simulink library "MotionPlanner_Library"  (R2025b)
settings: Solver=VariableStepAuto  StartTime=0.0  StopTime=10.0  RelTol=1e-3
values from neighbouring files (symbols this model uses):
  structMotionPlannerOut = struct()    [MotionPlanner_CreateExternalData.m]    (also in MotionPlanner_ExternalData.sldd = 0.0
                        0.0
                    
       )
undefined symbols (not defined in the file or in its folder): enable, finalPose, initialStateAndInput, originLLA, reset, samplingBoxCenterPose, samplingBoxDimension, sequentialPlanner, timestamp, verticesStaticObstacles
libraries: AVE_Library x7, MPSV x4, simulink x3, GenericTarget x1, simulink_extras x1
settings Model: Creator=damerius  LastModifiedBy=Scythe

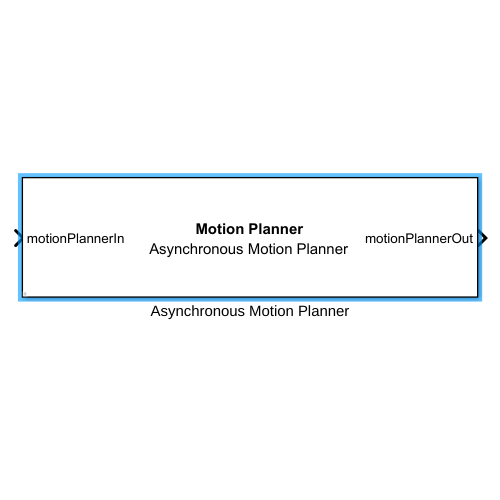
[thumbnail: Simulink's stored preview of the top-level diagram]
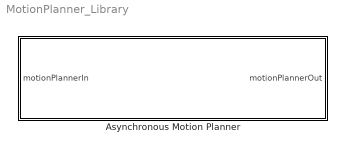
== system MotionPlanner_Library ==
  Asynchronous Motion Planner : Subsystem  mask{priorityWorkerThread=40, mpsvCPUCoresToUse=int32(0:7), sampletime=-1}
      mask prompts: priorityWorkerThread "Worker thread priority (1: low, 99: high):"; mpsvCPUCoresToUse "CPU cores on which the thread is eligible to run, e.g. [0,1,2,3] ([] to ignore):"; sampletime "Sample time (-1 for inherited):"
      mask help: Solves the motion planning problem in an asynchronous manner using parallel computing. The whole planner runs in a separate worker thread. Each time this block is executed, it passes data to the worker thread and fetches the latest results from it.
      mask DialogControl DescGroupVar Prompt: Asynchronous Motion Planner
      mask Display:
      | % Get dimension of block
      | pos = get_param(gcb, 'Position');
      | width = pos(3) - pos(1);
      | height = pos(4) - pos(2);
      | 
      | % Block title
      | text(0.5*width,0.5*height, '{\bfMotion Planner}','horizontalAlignment','center','verticalAlignment','bottom','texmode','on');
      | text(0.5*width,0.5*height, 'Asynchronous Motion Planner','horizontalAlignment','center','verticalAlignment','top','texmode','on');

== system MotionPlanner_Library/Asynchronous Motion Planner ==
  motionPlannerIn : Inport  OutDataTypeStr=Bus: busMotionPlannerIn  SampleTime=sampletime
  Asynchronous Motion Planner : Subsystem  TreatAsAtomicUnit=on
  Bus Selector : BusSelector  OutputSignals=parameter
  Planning Problem Generator : Subsystem
  Unit Delay : UnitDelay  SampleTime=sampletime  HasFrameUpgradeWarning=on
  check for automatic reset : Subsystem
  make output struct : Subsystem
  motionPlannerOut : Outport  OutDataTypeStr=Bus: busMotionPlannerOut  SampleTime=sampletime
  wires:
  make output struct/1(output) -> motionPlannerOut/1
  check for automatic reset/1(resetPlanner) -> Asynchronous Motion Planner/3(resetPlanner)
  Planning Problem Generator/1(planningProblem) -> Asynchronous Motion Planner/1(planningProblem)
  Asynchronous Motion Planner/1(motionPlanner) -> Unit Delay/1, make output struct/1(motionPlanner)
  Unit Delay/1 -> check for automatic reset/2(previousMotionPlanner)
  motionPlannerIn/1 -> check for automatic reset/1(input), Bus Selector/1, Planning Problem Generator/1(input)
  Bus Selector/1 -> Asynchronous Motion Planner/2(inputParameter)  "<parameter>"

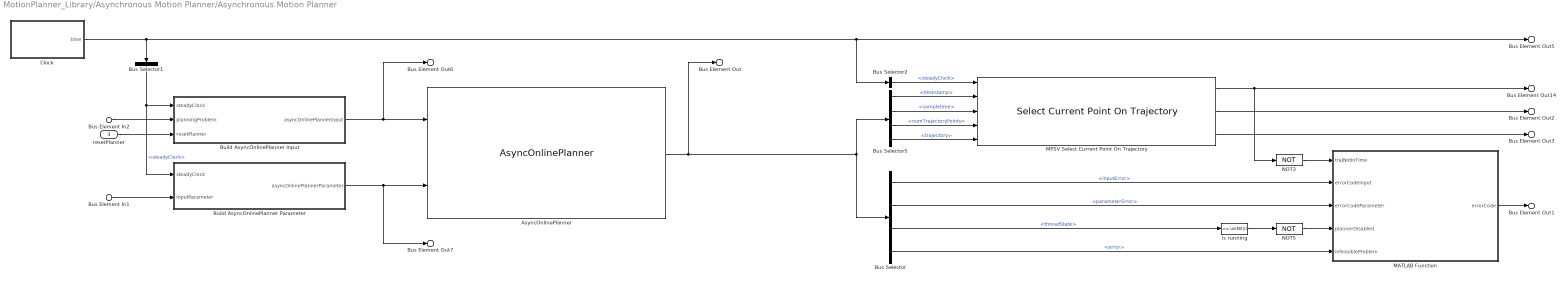
== system MotionPlanner_Library/Asynchronous Motion Planner/Asynchronous Motion Planner ==
  Bus Element In2 : Inport  PortName=planningProblem
  Bus Element In1 : Inport  Port=2  PortName=inputParameter
  resetPlanner : Inport  Port=3
  AsyncOnlinePlanner : MPSV/AsyncOnlinePlanner  pathMaxNumNodes=200  pathMaxNumSamples=1000000  motionMaxNumNodes=200  motionMaxNumSamples=1000000  threadPriority=priorityWorkerThread  cpuCoreIDs=mpsvCPUCoresToUse  ompNumThreads=numel(mpsvCPUCoresToUse) - 1  ompDynamic=0
      settings: SourceProductName=MPSV - Motion Planner for Surface Vehicles
  Build AsyncOnlinePlanner Input : Subsystem  Priority=2  TreatAsAtomicUnit=on
  Build AsyncOnlinePlanner Parameter : Subsystem  Priority=3  TreatAsAtomicUnit=on
  Bus Selector : BusSelector  OutputSignals=inputError,parameterError,threadState,error
  Bus Selector1 : BusSelector  OutputSignals=steadyClock
  Bus Selector2 : BusSelector  OutputSignals=steadyClock
  Bus Selector5 : BusSelector  OutputSignals=timestamp,sampletime,numTrajectoryPoints,trajectory
  Clock : Subsystem  Priority=1  TreatAsAtomicUnit=on  SystemSampleTime=sampletime
  MATLAB Function : MATLAB Function  TreatAsAtomicUnit=on
  MPSV Select Current Point On Trajectory : MPSV/Select Current Point On Trajectory
      settings: SourceProductName=MPSV - Motion Planner for Surface Vehicles
  NOT3 : Logic  Operator=NOT  AllPortsSameDT=off  OutDataTypeStr=boolean
  NOT5 : Logic  Operator=NOT  AllPortsSameDT=off  OutDataTypeStr=boolean
  is running : simulink/Logic and Bit Operations/Compare To Constant  relop===  const=uint8(2)  OutDataTypeStr=boolean
  Bus Element Out5 : Outport  PortName=motionPlanner  Element=time
  Bus Element Out : Outport  PortName=motionPlanner  Element=asyncOnlinePlannerOutput
  Bus Element Out14 : Outport  PortName=motionPlanner  Element=trajectoryPointSelector.success
  Bus Element Out2 : Outport  PortName=motionPlanner  Element=trajectoryPointSelector.currentPoint
  Bus Element Out3 : Outport  PortName=motionPlanner  Element=trajectoryPointSelector.remainingTrajectoryDuration
  Bus Element Out6 : Outport  PortName=motionPlanner  Element=asyncOnlinePlannerInput
  Bus Element Out7 : Outport  PortName=motionPlanner  Element=asyncOnlinePlannerParameter
  Bus Element Out1 : Outport  PortName=motionPlanner  Element=errorCode
  wires:
  MATLAB Function/1(errorCode) -> Bus Element Out1/1
  NOT3/1 -> MATLAB Function/1(trajNotInTime)
  Bus Selector/2 -> MATLAB Function/3(errorCodeParameter)  "<parameterError>"
  Bus Selector/1 -> MATLAB Function/2(errorCodeInput)  "<inputError>"
  resetPlanner/1 -> Build AsyncOnlinePlanner Input/3(resetPlanner)
  Bus Selector/4 -> MATLAB Function/5(infeasibleProblem)  "<error>"
  Bus Selector/3 -> is running/1  "<threadState>"
  Build AsyncOnlinePlanner Input/1(asyncOnlinePlannerInput) -> Bus Element Out6/1, AsyncOnlinePlanner/1
  AsyncOnlinePlanner/1 -> Bus Element Out/1, Bus Selector/1, Bus Selector5/1
  Bus Selector5/3 -> MPSV Select Current Point On Trajectory/4  "<numTrajectoryPoints>"
  Bus Selector5/1 -> MPSV Select Current Point On Trajectory/2  "<timestamp>"
  Bus Selector5/4 -> MPSV Select Current Point On Trajectory/5  "<trajectory>"
  Build AsyncOnlinePlanner Parameter/1(asyncOnlinePlannerParameter) -> Bus Element Out7/1, AsyncOnlinePlanner/2
  Bus Selector5/2 -> MPSV Select Current Point On Trajectory/3  "<sampletime>"
  MPSV Select Current Point On Trajectory/1 -> NOT3/1, Bus Element Out14/1
  MPSV Select Current Point On Trajectory/2 -> Bus Element Out2/1
  MPSV Select Current Point On Trajectory/3 -> Bus Element Out3/1
  Bus Element In2/1 -> Build AsyncOnlinePlanner Input/2(planningProblem)
  Bus Element In1/1 -> Build AsyncOnlinePlanner Parameter/2(inputParameter)
  is running/1 -> NOT5/1
  NOT5/1 -> MATLAB Function/4(plannerDisabled)
  Clock/1(time) -> Bus Selector2/1, Bus Element Out5/1, Bus Selector1/1
  Bus Selector1/1 -> Build AsyncOnlinePlanner Input/1(steadyClock), Build AsyncOnlinePlanner Parameter/1(steadyClock)  "<steadyClock>"
  Bus Selector2/1 -> MPSV Select Current Point On Trajectory/1  "<steadyClock>"

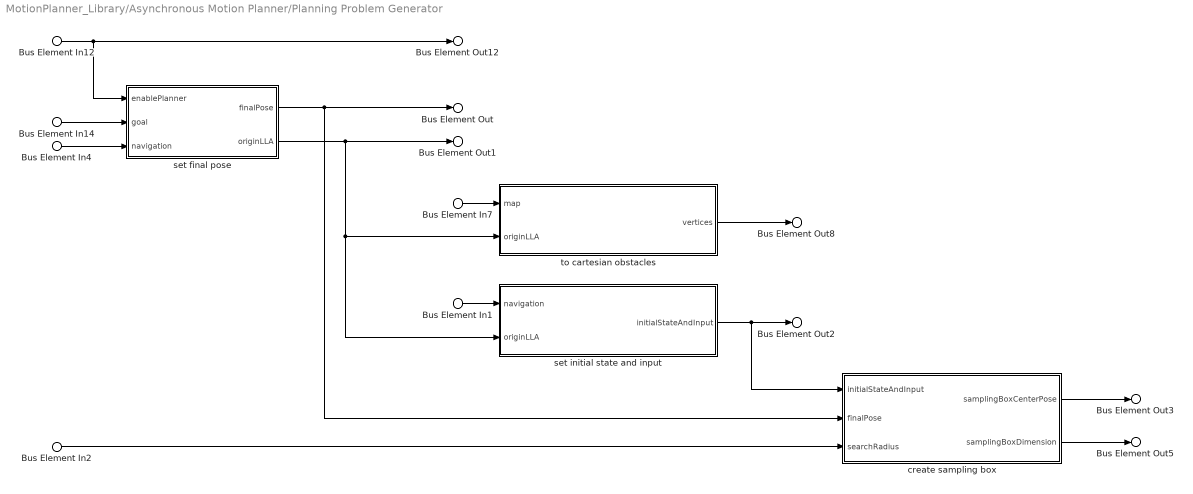
== system MotionPlanner_Library/Asynchronous Motion Planner/Planning Problem Generator ==
  Bus Element In14 : Inport  PortName=input  Element=goal
  Bus Element In7 : Inport  PortName=input  Element=map
  Bus Element In12 : Inport  PortName=input  Element=enablePlanner
  Bus Element In4 : Inport  PortName=input  Element=navigation
  Bus Element In1 : Inport  PortName=input  Element=navigation
  Bus Element In2 : Inport  PortName=input  Element=parameter.searchRadius
  create sampling box : Subsystem
  set final pose : Subsystem
  set initial state and input : Subsystem
  to cartesian obstacles : Subsystem
  Bus Element Out12 : Outport  PortName=planningProblem  Element=enablePlanner
  Bus Element Out1 : Outport  PortName=planningProblem  Element=originLLA
  Bus Element Out2 : Outport  PortName=planningProblem  Element=initialStateAndInput
  Bus Element Out : Outport  PortName=planningProblem  Element=finalPose
  Bus Element Out3 : Outport  PortName=planningProblem  Element=samplingBoxCenterPose
  Bus Element Out5 : Outport  PortName=planningProblem  Element=samplingBoxDimension
  Bus Element Out8 : Outport  PortName=planningProblem  Element=staticObstacles.vertices
  wires:
  Bus Element In12/1 -> Bus Element Out12/1, set final pose/1(enablePlanner)
  to cartesian obstacles/1(vertices) -> Bus Element Out8/1
  Bus Element In7/1 -> to cartesian obstacles/1(map)
  create sampling box/2(samplingBoxDimension) -> Bus Element Out5/1
  create sampling box/1(samplingBoxCenterPose) -> Bus Element Out3/1
  Bus Element In2/1 -> create sampling box/3(searchRadius)
  set initial state and input/1(initialStateAndInput) -> create sampling box/1(initialStateAndInput), Bus Element Out2/1
  set final pose/2(originLLA) -> Bus Element Out1/1, set initial state and input/2(originLLA), to cartesian obstacles/2(originLLA)
  set final pose/1(finalPose) -> Bus Element Out/1, create sampling box/2(finalPose)
  Bus Element In14/1 -> set final pose/2(goal)
  Bus Element In4/1 -> set final pose/3(navigation)
  Bus Element In1/1 -> set initial state and input/1(navigation)

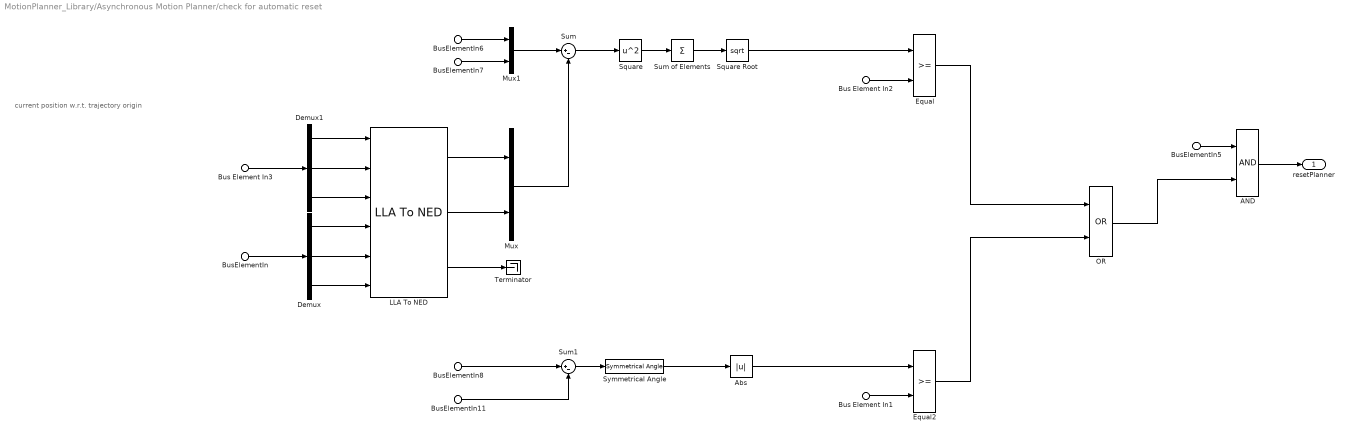
== system MotionPlanner_Library/Asynchronous Motion Planner/check for automatic reset ==
  note: current position w.r.t. trajectory origin
  Bus Element In3 : Inport  PortName=input  Element=navigation.positionLLA
  BusElementIn11 : Inport  PortName=input  Element=navigation.orientationYaw
  Bus Element In2 : Inport  PortName=input  Element=maxDeviationToReset.position
  Bus Element In1 : Inport  PortName=input  Element=maxDeviationToReset.heading
  BusElementIn : Inport  Port=2  PortName=previousMotionPlanner  Element=asyncOnlinePlannerOutput.originLLA
  BusElementIn5 : Inport  Port=2  PortName=previousMotionPlanner  Element=trajectoryPointSelector.success
  BusElementIn6 : Inport  Port=2  PortName=previousMotionPlanner  Element=trajectoryPointSelector.currentPoint.stateInterpolated.positionNorth
  BusElementIn7 : Inport  Port=2  PortName=previousMotionPlanner  Element=trajectoryPointSelector.currentPoint.stateInterpolated.positionEast
  BusElementIn8 : Inport  Port=2  PortName=previousMotionPlanner  Element=trajectoryPointSelector.currentPoint.stateInterpolated.orientationYaw
  AND : Logic  AllPortsSameDT=off  OutDataTypeStr=boolean
  Abs : Abs  SaturateOnIntegerOverflow=off
  Demux : Demux  Outputs=3
  Demux1 : Demux  Outputs=3
  Equal : RelationalOperator  OutDataTypeStr=boolean  RndMeth=Simplest  InputSameDT=off
  Equal2 : RelationalOperator  OutDataTypeStr=boolean  RndMeth=Simplest  InputSameDT=off
  LLA To NED : AVE_Library/Essential/Transformation/LLA To NED
      settings: SourceProductName=AVE - Autonomous Vehicle Control Toolbox
  Mux : Mux  Inputs=2
  Mux1 : Mux  Inputs=2
  OR : Logic  Operator=OR  AllPortsSameDT=off  OutDataTypeStr=boolean
  Square : Math  Operator=square
  Square Root : Sqrt
  Sum : Sum  Inputs=|+-
  Sum of Elements : Sum  Inputs=+
  Sum1 : Sum  Inputs=|+-
  Symmetrical Angle : AVE_Library/Essential/Symmetrical Angle
      settings: SourceProductName=AVE - Autonomous Vehicle Control Toolbox
  Terminator : Terminator
  resetPlanner : Outport
  wires:
  Demux1/3 -> LLA To NED/3
  Demux1/2 -> LLA To NED/2
  Demux1/1 -> LLA To NED/1
  Bus Element In3/1 -> Demux1/1
  BusElementIn/1 -> Demux/1
  Demux/1 -> LLA To NED/4
  Demux/2 -> LLA To NED/5
  Demux/3 -> LLA To NED/6
  LLA To NED/3 -> Terminator/1
  LLA To NED/2 -> Mux/2
  LLA To NED/1 -> Mux/1
  BusElementIn6/1 -> Mux1/1
  BusElementIn7/1 -> Mux1/2
  Mux1/1 -> Sum/1
  Mux/1 -> Sum/2
  Sum/1 -> Square/1
  Square/1 -> Sum of Elements/1
  Sum of Elements/1 -> Square Root/1
  BusElementIn8/1 -> Sum1/1
  BusElementIn11/1 -> Sum1/2
  Sum1/1 -> Symmetrical Angle/1
  Symmetrical Angle/1 -> Abs/1
  BusElementIn5/1 -> AND/1
  AND/1 -> resetPlanner/1
  OR/1 -> AND/2
  Square Root/1 -> Equal/1
  Bus Element In2/1 -> Equal/2
  Abs/1 -> Equal2/1
  Bus Element In1/1 -> Equal2/2
  Equal/1 -> OR/1
  Equal2/1 -> OR/2

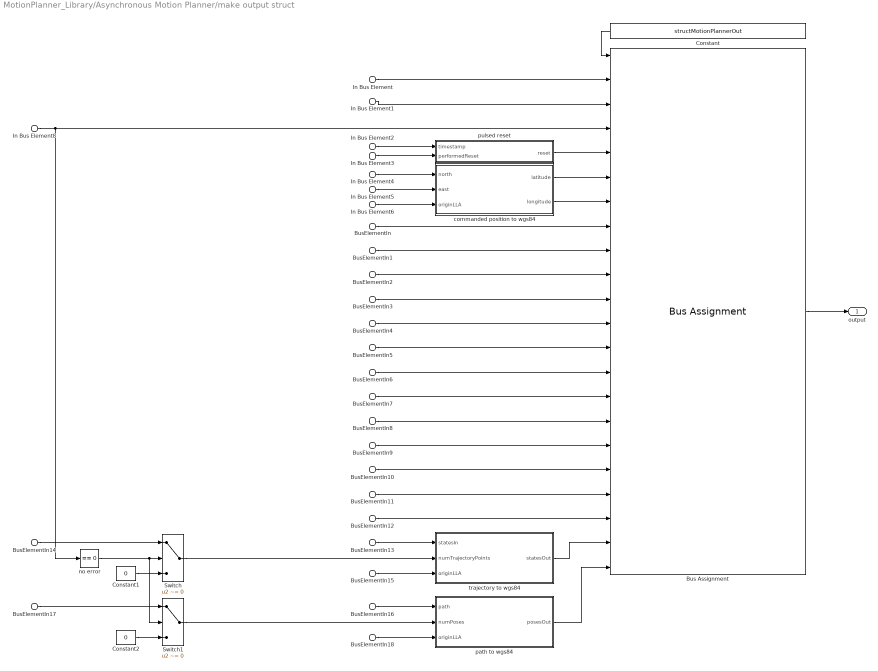
== system MotionPlanner_Library/Asynchronous Motion Planner/make output struct ==
  In Bus Element : Inport  PortName=motionPlanner  Element=time.timestampUTC
  In Bus Element1 : Inport  PortName=motionPlanner  Element=time.steadyClock
  In Bus Element3 : Inport  PortName=motionPlanner  Element=asyncOnlinePlannerOutput.performedReset
  In Bus Element6 : Inport  PortName=motionPlanner  Element=asyncOnlinePlannerOutput.originLLA
  BusElementIn15 : Inport  PortName=motionPlanner  Element=asyncOnlinePlannerOutput.originLLA
  BusElementIn18 : Inport  PortName=motionPlanner  Element=asyncOnlinePlannerOutput.originLLA
  BusElementIn11 : Inport  PortName=motionPlanner  Element=asyncOnlinePlannerOutput.timestamp
  In Bus Element2 : Inport  PortName=motionPlanner  Element=asyncOnlinePlannerOutput.timestamp
  BusElementIn12 : Inport  PortName=motionPlanner  Element=asyncOnlinePlannerOutput.sampletime
  BusElementIn13 : Inport  PortName=motionPlanner  Element=asyncOnlinePlannerOutput.trajectory
  BusElementIn14 : Inport  PortName=motionPlanner  Element=asyncOnlinePlannerOutput.numTrajectoryPoints
  BusElementIn16 : Inport  PortName=motionPlanner  Element=asyncOnlinePlannerOutput.pathPlanner.path
  BusElementIn17 : Inport  PortName=motionPlanner  Element=asyncOnlinePlannerOutput.pathPlanner.numPoses
  In Bus Element4 : Inport  PortName=motionPlanner  Element=trajectoryPointSelector.currentPoint.stateInterpolated.positionNorth
  In Bus Element5 : Inport  PortName=motionPlanner  Element=trajectoryPointSelector.currentPoint.stateInterpolated.positionEast
  BusElementIn : Inport  PortName=motionPlanner  Element=trajectoryPointSelector.currentPoint.stateInterpolated.orientationYaw
  BusElementIn1 : Inport  PortName=motionPlanner  Element=trajectoryPointSelector.currentPoint.stateInterpolated.velocityU
  BusElementIn2 : Inport  PortName=motionPlanner  Element=trajectoryPointSelector.currentPoint.stateInterpolated.velocityV
  BusElementIn3 : Inport  PortName=motionPlanner  Element=trajectoryPointSelector.currentPoint.stateInterpolated.velocityR
  BusElementIn4 : Inport  PortName=motionPlanner  Element=trajectoryPointSelector.currentPoint.stateInterpolated.tauX
  BusElementIn5 : Inport  PortName=motionPlanner  Element=trajectoryPointSelector.currentPoint.stateInterpolated.tauY
  BusElementIn6 : Inport  PortName=motionPlanner  Element=trajectoryPointSelector.currentPoint.stateInterpolated.tauN
  BusElementIn7 : Inport  PortName=motionPlanner  Element=trajectoryPointSelector.currentPoint.controlInputZeroOrderHold.commandedTauX
  BusElementIn8 : Inport  PortName=motionPlanner  Element=trajectoryPointSelector.currentPoint.controlInputZeroOrderHold.commandedTauY
  BusElementIn9 : Inport  PortName=motionPlanner  Element=trajectoryPointSelector.currentPoint.controlInputZeroOrderHold.commandedTauN
  BusElementIn10 : Inport  PortName=motionPlanner  Element=trajectoryPointSelector.remainingTrajectoryDuration
  In Bus Element8 : Inport  PortName=motionPlanner  Element=errorCode
  Bus Assignment : BusAssignment  AssignedSignals=time.timestampUTC,time.steadyClock,errorCode,performedReset,controlCommand.commandedState.positionLatitude,controlCommand.commandedState.positionLongitude,controlCommand.commandedState.orientationYaw,controlCommand.commandedState.velocityU,controlCommand.commandedState.velocityV,controlCommand.commandedState.velocityR,controlCommand.commandedState.tauX,controlCommand.commandedState.tauY,controlCommand.commandedState.tauN,controlCommand.commandedInput.tauX,controlCommand.commandedInput.tauY,controlCommand.commandedInput.tauN,controlCommand.remainingTrajectoryDuration,trajectory.timestampSteadyClock,trajectory.sampletime,trajectory.states,path.poses
  Constant : Constant  Value=structMotionPlannerOut  OutDataTypeStr=Bus: busMotionPlannerOut
  Constant1 : Constant  Value=0  OutDataTypeStr=uint16
  Constant2 : Constant  Value=0  OutDataTypeStr=uint16
  Switch : Switch  Criteria=u2 ~= 0  SaturateOnIntegerOverflow=off  InputSameDT=off
  Switch1 : Switch  Criteria=u2 ~= 0  SaturateOnIntegerOverflow=off  InputSameDT=off
  commanded position to wgs84 : Subsystem
  no error : simulink/Logic and Bit Operations/Compare To Zero  relop===  OutDataTypeStr=boolean
  path to wgs84 : Subsystem
  pulsed reset : Subsystem
  trajectory to wgs84 : Subsystem
  output : Outport  OutDataTypeStr=Bus: busMotionPlannerOut
  wires:
  no error/1 -> Switch/2, Switch1/2
  Constant2/1 -> Switch1/3
  Constant1/1 -> Switch/3
  BusElementIn17/1 -> Switch1/1
  BusElementIn14/1 -> Switch/1
  path to wgs84/1(posesOut) -> Bus Assignment/22
  BusElementIn18/1 -> path to wgs84/3(originLLA)
  Switch1/1 -> path to wgs84/2(numPoses)
  BusElementIn16/1 -> path to wgs84/1(path)
  BusElementIn15/1 -> trajectory to wgs84/3(originLLA)
  Switch/1 -> trajectory to wgs84/2(numTrajectoryPoints)
  BusElementIn13/1 -> trajectory to wgs84/1(statesIn)
  trajectory to wgs84/1(statesOut) -> Bus Assignment/21
  BusElementIn12/1 -> Bus Assignment/20
  BusElementIn11/1 -> Bus Assignment/19
  BusElementIn10/1 -> Bus Assignment/18
  BusElementIn9/1 -> Bus Assignment/17
  BusElementIn8/1 -> Bus Assignment/16
  BusElementIn7/1 -> Bus Assignment/15
  BusElementIn6/1 -> Bus Assignment/14
  BusElementIn5/1 -> Bus Assignment/13
  BusElementIn4/1 -> Bus Assignment/12
  BusElementIn3/1 -> Bus Assignment/11
  BusElementIn2/1 -> Bus Assignment/10
  BusElementIn1/1 -> Bus Assignment/9
  BusElementIn/1 -> Bus Assignment/8
  In Bus Element6/1 -> commanded position to wgs84/3(originLLA)
  In Bus Element5/1 -> commanded position to wgs84/2(east)
  In Bus Element4/1 -> commanded position to wgs84/1(north)
  commanded position to wgs84/2(longitude) -> Bus Assignment/7
  commanded position to wgs84/1(latitude) -> Bus Assignment/6
  In Bus Element8/1 -> Bus Assignment/4, no error/1
  In Bus Element3/1 -> pulsed reset/2(performedReset)
  In Bus Element1/1 -> Bus Assignment/3
  In Bus Element/1 -> Bus Assignment/2
  Bus Assignment/1 -> output/1
  Constant/1 -> Bus Assignment/1
  In Bus Element2/1 -> pulsed reset/1(timestamp)
  pulsed reset/1(reset) -> Bus Assignment/5

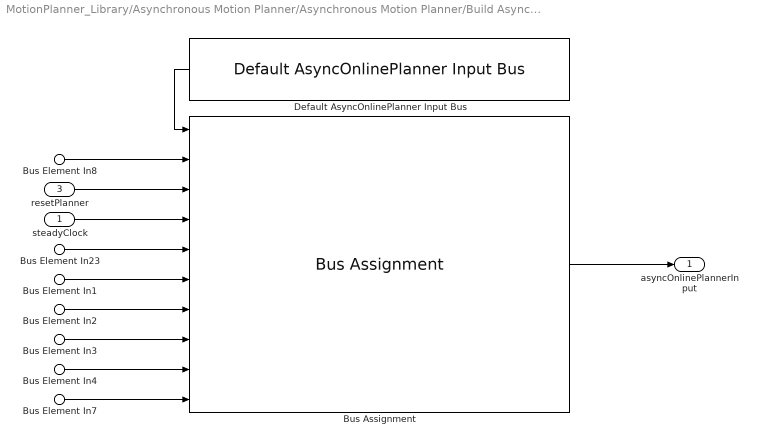
== system MotionPlanner_Library/Asynchronous Motion Planner/Asynchronous Motion Planner/Build AsyncOnlinePlanner Input ==
  steadyClock : Inport
  Bus Element In23 : Inport  Port=2  PortName=planningProblem  Element=originLLA
  Bus Element In1 : Inport  Port=2  PortName=planningProblem  Element=initialStateAndInput
  Bus Element In2 : Inport  Port=2  PortName=planningProblem  Element=finalPose
  Bus Element In3 : Inport  Port=2  PortName=planningProblem  Element=samplingBoxCenterPose
  Bus Element In4 : Inport  Port=2  PortName=planningProblem  Element=samplingBoxDimension
  Bus Element In7 : Inport  Port=2  PortName=planningProblem  Element=staticObstacles.vertices
  Bus Element In8 : Inport  Port=2  PortName=planningProblem  Element=enablePlanner
  resetPlanner : Inport  Port=3
  Bus Assignment : BusAssignment  AssignedSignals=enable,reset,timestamp,originLLA,initialStateAndInput,finalPose,samplingBoxCenterPose,samplingBoxDimension,verticesStaticObstacles
  Default AsyncOnlinePlanner Input Bus : MPSV/Default AsyncOnlinePlanner Input Bus
      settings: SourceProductName=MPSV - Motion Planner for Surface Vehicles
  asyncOnlinePlannerInput : Outport
  wires:
  resetPlanner/1 -> Bus Assignment/3
  Bus Element In8/1 -> Bus Assignment/2
  Bus Element In7/1 -> Bus Assignment/10
  Bus Element In4/1 -> Bus Assignment/9
  Bus Element In3/1 -> Bus Assignment/8
  Bus Element In2/1 -> Bus Assignment/7
  Bus Element In1/1 -> Bus Assignment/6
  Bus Element In23/1 -> Bus Assignment/5
  Default AsyncOnlinePlanner Input Bus/1 -> Bus Assignment/1
  Bus Assignment/1 -> asyncOnlinePlannerInput/1
  steadyClock/1 -> Bus Assignment/4

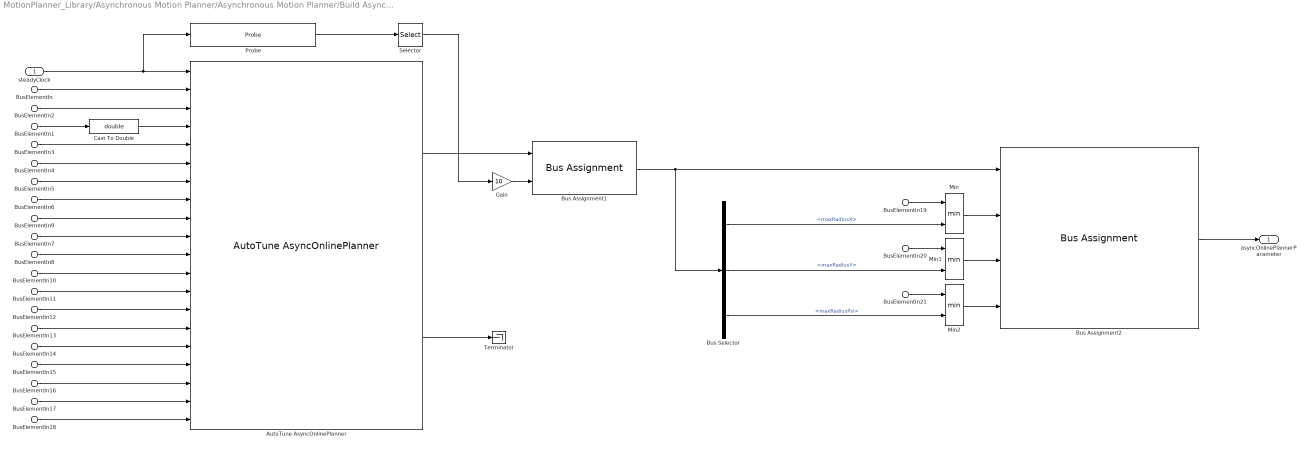
== system MotionPlanner_Library/Asynchronous Motion Planner/Asynchronous Motion Planner/Build AsyncOnlinePlanner Parameter ==
  steadyClock : Inport
  BusElementIn : Inport  Port=2  PortName=inputParameter  Element=controlEffort
  BusElementIn1 : Inport  Port=2  PortName=inputParameter  Element=geometry.verticesVehicleShape
  BusElementIn3 : Inport  Port=2  PortName=inputParameter  Element=geometry.collisionCheckMaxPositionDeviation
  BusElementIn4 : Inport  Port=2  PortName=inputParameter  Element=geometry.collisionCheckMaxAngleDeviation
  BusElementIn5 : Inport  Port=2  PortName=inputParameter  Element=model.matF
  BusElementIn6 : Inport  Port=2  PortName=inputParameter  Element=model.matB
  BusElementIn7 : Inport  Port=2  PortName=inputParameter  Element=model.vecTimeconstantsXYN
  BusElementIn8 : Inport  Port=2  PortName=inputParameter  Element=model.vecTimeconstantsInput
  BusElementIn9 : Inport  Port=2  PortName=inputParameter  Element=model.vecSatXYN
  BusElementIn10 : Inport  Port=2  PortName=inputParameter  Element=timing.trajectorySampletime
  BusElementIn11 : Inport  Port=2  PortName=inputParameter  Element=timing.maxComputationTimePath
  BusElementIn12 : Inport  Port=2  PortName=inputParameter  Element=timing.maxComputationTimeMotion
  BusElementIn13 : Inport  Port=2  PortName=inputParameter  Element=metric.weightPsi
  BusElementIn14 : Inport  Port=2  PortName=inputParameter  Element=metric.weightSway
  BusElementIn15 : Inport  Port=2  PortName=inputParameter  Element=metric.weightReverseScale
  BusElementIn16 : Inport  Port=2  PortName=inputParameter  Element=metric.weightReverseDecay
  BusElementIn17 : Inport  Port=2  PortName=inputParameter  Element=metric.distanceScale
  BusElementIn18 : Inport  Port=2  PortName=inputParameter  Element=metric.distanceDecay
  BusElementIn2 : Inport  Port=2  PortName=inputParameter  Element=explorePath.desiredRadiusX
  BusElementIn19 : Inport  Port=2  PortName=inputParameter  Element=explorePath.maxRadiusX
  BusElementIn20 : Inport  Port=2  PortName=inputParameter  Element=explorePath.maxRadiusY
  BusElementIn21 : Inport  Port=2  PortName=inputParameter  Element=explorePath.maxRadiusPsi
  AutoTune AsyncOnlinePlanner : MPSV/AutoTune AsyncOnlinePlanner  timeoutInput=1  periodGoalSampling=30
      settings: SourceProductName=MPSV - Motion Planner for Surface Vehicles
  Bus Assignment1 : BusAssignment  AssignedSignals=timeoutInput
  Bus Assignment2 : BusAssignment  AssignedSignals=sequentialPlanner.motionPlanner.controller.maxRadiusX,sequentialPlanner.motionPlanner.controller.maxRadiusY,sequentialPlanner.motionPlanner.controller.maxRadiusPsi
  Bus Selector : BusSelector  OutputSignals=sequentialPlanner.motionPlanner.controller.maxRadiusX,sequentialPlanner.motionPlanner.controller.maxRadiusY,sequentialPlanner.motionPlanner.controller.maxRadiusPsi
  Cast To Double : DataTypeConversion  OutDataTypeStr=double  SaturateOnIntegerOverflow=off  RndMeth=Floor
  Gain : Gain  Gain=10
  Min : MinMax  Inputs=2
  Min1 : MinMax  Inputs=2
  Min2 : MinMax  Inputs=2
  Probe : Probe  ProbeWidth=off  ProbeComplexSignal=off
  Selector : Selector  InputPortWidth=2  IndexOptions=Index vector (dialog)  Indices=1  OutputSizes=1
  Terminator : Terminator
  asyncOnlinePlannerParameter : Outport
  wires:
  AutoTune AsyncOnlinePlanner/1 -> Bus Assignment1/1
  AutoTune AsyncOnlinePlanner/2 -> Terminator/1
  steadyClock/1 -> Probe/1, AutoTune AsyncOnlinePlanner/1
  Bus Assignment1/1 -> Bus Selector/1, Bus Assignment2/1
  BusElementIn1/1 -> Cast To Double/1
  Gain/1 -> Bus Assignment1/2
  Probe/1 -> Selector/1
  Selector/1 -> Gain/1
  BusElementIn/1 -> AutoTune AsyncOnlinePlanner/2
  BusElementIn2/1 -> AutoTune AsyncOnlinePlanner/3
  Cast To Double/1 -> AutoTune AsyncOnlinePlanner/4
  BusElementIn3/1 -> AutoTune AsyncOnlinePlanner/5
  BusElementIn4/1 -> AutoTune AsyncOnlinePlanner/6
  BusElementIn5/1 -> AutoTune AsyncOnlinePlanner/7
  BusElementIn6/1 -> AutoTune AsyncOnlinePlanner/8
  BusElementIn9/1 -> AutoTune AsyncOnlinePlanner/9
  BusElementIn7/1 -> AutoTune AsyncOnlinePlanner/10
  BusElementIn8/1 -> AutoTune AsyncOnlinePlanner/11
  BusElementIn10/1 -> AutoTune AsyncOnlinePlanner/12
  BusElementIn11/1 -> AutoTune AsyncOnlinePlanner/13
  BusElementIn12/1 -> AutoTune AsyncOnlinePlanner/14
  BusElementIn13/1 -> AutoTune AsyncOnlinePlanner/15
  BusElementIn14/1 -> AutoTune AsyncOnlinePlanner/16
  BusElementIn15/1 -> AutoTune AsyncOnlinePlanner/17
  BusElementIn16/1 -> AutoTune AsyncOnlinePlanner/18
  BusElementIn17/1 -> AutoTune AsyncOnlinePlanner/19
  BusElementIn18/1 -> AutoTune AsyncOnlinePlanner/20
  Bus Assignment2/1 -> asyncOnlinePlannerParameter/1
  Min/1 -> Bus Assignment2/2
  Min1/1 -> Bus Assignment2/3
  Min2/1 -> Bus Assignment2/4
  BusElementIn19/1 -> Min/1
  BusElementIn20/1 -> Min1/1
  BusElementIn21/1 -> Min2/1
  Bus Selector/1 -> Min/2  "<maxRadiusX>"
  Bus Selector/2 -> Min1/2  "<maxRadiusY>"
  Bus Selector/3 -> Min2/2  "<maxRadiusPsi>"

== system MotionPlanner_Library/Asynchronous Motion Planner/Asynchronous Motion Planner/Clock ==
  note: inherit sampletime from atomic subsystem
  UTC Timestamp : GenericTarget/Time/UTC Timestamp  SampleTime=-1
      settings: SourceProductName=Generic Target
  counter based steady clock : DigitalClock  SampleTime=-1
  Out Bus Element : Outport  PortName=time  Element=steadyClock
  Out Bus Element1 : Outport  PortName=time  Element=timestampUTC
  wires:
  counter based steady clock/1 -> Out Bus Element/1
  UTC Timestamp/1 -> Out Bus Element1/1

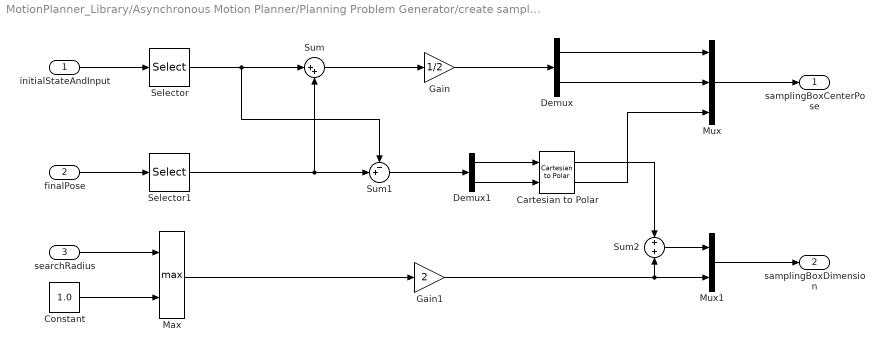
== system MotionPlanner_Library/Asynchronous Motion Planner/Planning Problem Generator/create sampling box ==
  initialStateAndInput : Inport
  finalPose : Inport  Port=2
  searchRadius : Inport  Port=3
  Cartesian to Polar : simulink_extras/Transformations/Cartesian to Polar
  Constant : Constant  Value=1.0
  Demux : Demux  Outputs=2
  Demux1 : Demux  Outputs=2
  Gain : Gain  Gain=1/2
  Gain1 : Gain  Gain=2
  Max : MinMax  Function=max  Inputs=2
  Mux : Mux  Inputs=3
  Mux1 : Mux  Inputs=2
  Selector : Selector  InputPortWidth=12  IndexOptions=Index vector (dialog)  Indices=[1 2]  OutputSizes=1
  Selector1 : Selector  InputPortWidth=3  IndexOptions=Index vector (dialog)  Indices=[1 2]  OutputSizes=1
  Sum : Sum  Inputs=|++
  Sum1 : Sum  Inputs=-+|
  Sum2 : Sum
  samplingBoxCenterPose : Outport
  samplingBoxDimension : Outport  Port=2
  wires:
  finalPose/1 -> Selector1/1
  initialStateAndInput/1 -> Selector/1
  Cartesian to Polar/1 -> Sum2/1
  Gain1/1 -> Mux1/2, Sum2/2
  Sum2/1 -> Mux1/1
  Cartesian to Polar/2 -> Mux/3
  Demux/2 -> Mux/2
  Demux/1 -> Mux/1
  Sum1/1 -> Demux1/1
  Demux1/1 -> Cartesian to Polar/1
  Demux1/2 -> Cartesian to Polar/2
  Gain/1 -> Demux/1
  Sum/1 -> Gain/1
  Mux1/1 -> samplingBoxDimension/1
  Mux/1 -> samplingBoxCenterPose/1
  Max/1 -> Gain1/1
  Selector1/1 -> Sum/2, Sum1/2
  Selector/1 -> Sum/1, Sum1/1
  searchRadius/1 -> Max/1
  Constant/1 -> Max/2

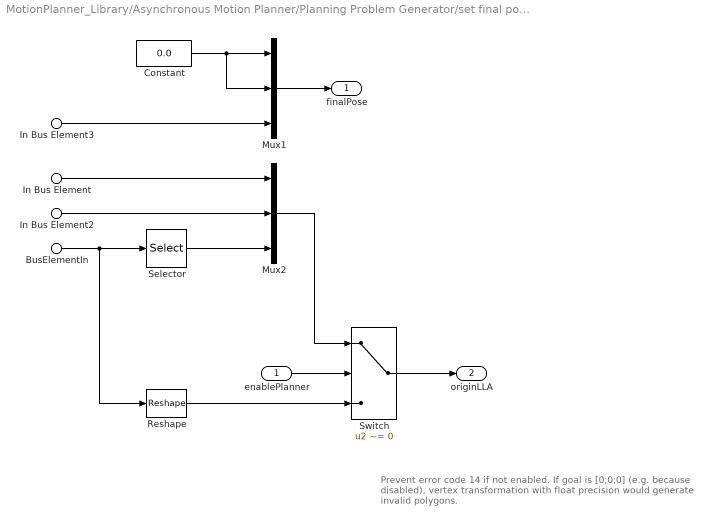
== system MotionPlanner_Library/Asynchronous Motion Planner/Planning Problem Generator/set final pose ==
  note: Prevent error code 14 if not enabled.
      | If goal is [0;0;0] (e.g. because disabled), vertex transformation with float precision would generate invalid polygons.
  enablePlanner : Inport
  In Bus Element : Inport  Port=2  PortName=goal  Element=positionLatitude
  In Bus Element2 : Inport  Port=2  PortName=goal  Element=positionLongitude
  In Bus Element3 : Inport  Port=2  PortName=goal  Element=orientationYaw
  BusElementIn : Inport  Port=3  PortName=navigation  Element=positionLLA
  Constant : Constant  Value=0.0
  Mux1 : Mux  Inputs=3
  Mux2 : Mux  Inputs=3
  Reshape : Reshape
  Selector : Selector  InputPortWidth=3  IndexOptions=Index vector (dialog)  Indices=3  OutputSizes=1
  Switch : Switch  Criteria=u2 ~= 0  SaturateOnIntegerOverflow=off  InputSameDT=off
  finalPose : Outport
  originLLA : Outport  Port=2
  wires:
  Reshape/1 -> Switch/3
  Switch/1 -> originLLA/1
  enablePlanner/1 -> Switch/2
  BusElementIn/1 -> Selector/1, Reshape/1
  Mux2/1 -> Switch/1
  In Bus Element3/1 -> Mux1/3
  Mux1/1 -> finalPose/1
  Constant/1 -> Mux1/1, Mux1/2
  In Bus Element/1 -> Mux2/1
  In Bus Element2/1 -> Mux2/2
  Selector/1 -> Mux2/3

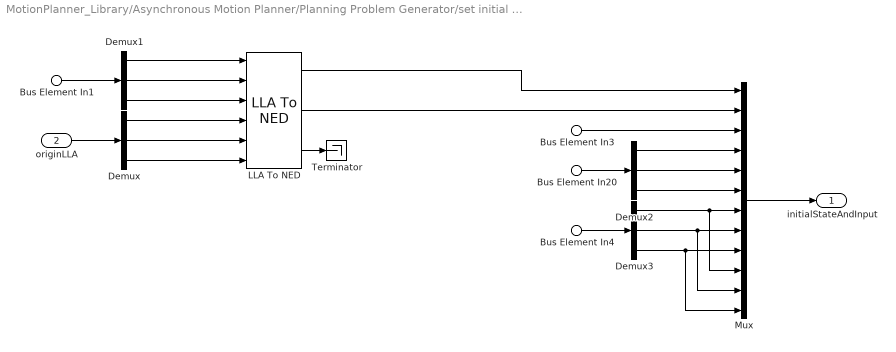
== system MotionPlanner_Library/Asynchronous Motion Planner/Planning Problem Generator/set initial state and input ==
  Bus Element In4 : Inport  PortName=navigation  Element=actualForceXYN
  Bus Element In3 : Inport  PortName=navigation  Element=orientationYaw
  Bus Element In20 : Inport  PortName=navigation  Element=velocityUVR
  Bus Element In1 : Inport  PortName=navigation  Element=positionLLA
  originLLA : Inport  Port=2
  Demux{,1..3} (4 alike) : Demux  Outputs=3
  LLA To NED : AVE_Library/Essential/Transformation/LLA To NED
      settings: SourceProductName=AVE - Autonomous Vehicle Control Toolbox
  Mux : Mux  Inputs=12
  Terminator : Terminator
  initialStateAndInput : Outport
  wires:
  Bus Element In4/1 -> Demux3/1
  Bus Element In20/1 -> Demux2/1
  Demux2/1 -> Mux/4
  Demux2/3 -> Mux/6
  Demux2/2 -> Mux/5
  Bus Element In1/1 -> Demux1/1
  Demux1/3 -> LLA To NED/3
  Demux1/2 -> LLA To NED/2
  Demux1/1 -> LLA To NED/1
  Demux/3 -> LLA To NED/6
  Demux/2 -> LLA To NED/5
  Demux/1 -> LLA To NED/4
  originLLA/1 -> Demux/1
  Mux/1 -> initialStateAndInput/1
  Bus Element In3/1 -> Mux/3
  LLA To NED/3 -> Terminator/1
  LLA To NED/1 -> Mux/1
  Demux3/3 -> Mux/9, Mux/12
  Demux3/2 -> Mux/8, Mux/11
  Demux3/1 -> Mux/7, Mux/10
  LLA To NED/2 -> Mux/2

== system MotionPlanner_Library/Asynchronous Motion Planner/Planning Problem Generator/to cartesian obstacles ==
  note: y = u1 + u2
  Bus Element In2 : Inport  PortName=map  Element=vertices
  BusElementIn : Inport  PortName=map  Element=originLLA
  originLLA : Inport  Port=2
  Demux1 : Demux  Outputs=3
  Demux2 : Demux  Outputs=3
  LLA To NED : AVE_Library/Essential/Transformation/LLA To NED
      settings: SourceProductName=AVE - Autonomous Vehicle Control Toolbox
  Mux : Mux  Inputs=2
  Reshape : Reshape  OutputDimensionality=Column vector (2-D)
  Terminator : Terminator
  add_matlab : MATLAB Function  TreatAsAtomicUnit=on
  vertices : Outport
  wires:
  BusElementIn/1 -> Demux2/1
  Demux2/3 -> LLA To NED/3
  Demux2/2 -> LLA To NED/2
  Demux2/1 -> LLA To NED/1
  Mux/1 -> Reshape/1
  LLA To NED/2 -> Mux/2
  LLA To NED/1 -> Mux/1
  LLA To NED/3 -> Terminator/1
  originLLA/1 -> Demux1/1
  Demux1/3 -> LLA To NED/6
  Demux1/2 -> LLA To NED/5
  Demux1/1 -> LLA To NED/4
  add_matlab/1(y) -> vertices/1
  Bus Element In2/1 -> add_matlab/1(u1)
  Reshape/1 -> add_matlab/2(u2)

== system MotionPlanner_Library/Asynchronous Motion Planner/make output struct/commanded position to wgs84 ==
  north : Inport
  east : Inport  Port=2
  originLLA : Inport  Port=3
  Demux : Demux  Outputs=3
  Ground : Ground
  NED To LLA : AVE_Library/Essential/Transformation/NED To LLA
      settings: SourceProductName=AVE - Autonomous Vehicle Control Toolbox
  Terminator : Terminator
  latitude : Outport
  longitude : Outport  Port=2
  wires:
  NED To LLA/1 -> latitude/1
  NED To LLA/2 -> longitude/1
  NED To LLA/3 -> Terminator/1
  north/1 -> NED To LLA/1
  east/1 -> NED To LLA/2
  Ground/1 -> NED To LLA/3
  Demux/3 -> NED To LLA/6
  Demux/2 -> NED To LLA/5
  Demux/1 -> NED To LLA/4
  originLLA/1 -> Demux/1

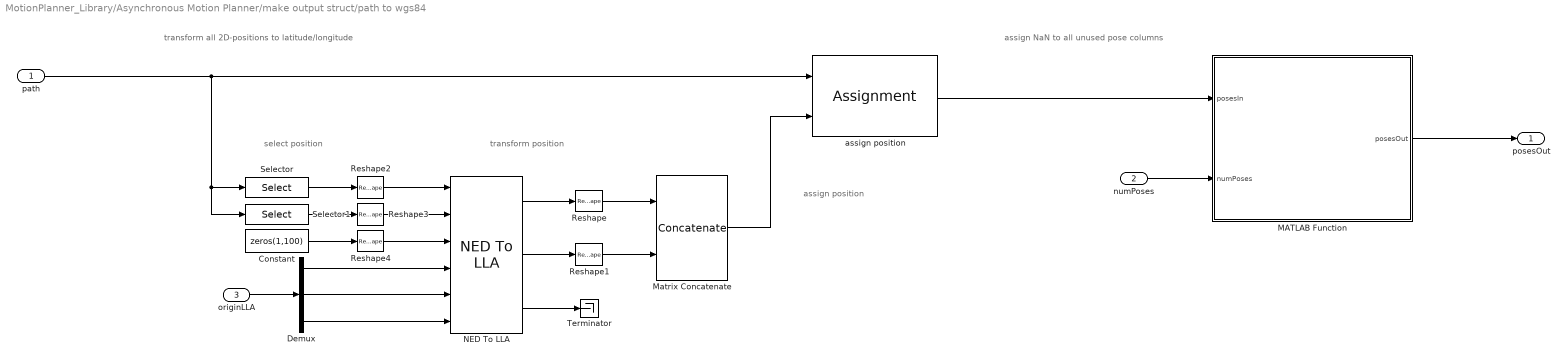
== system MotionPlanner_Library/Asynchronous Motion Planner/make output struct/path to wgs84 ==
  note: assign NaN to all unused pose columns
  note: assign position
  note: transform position
  note: transform all 2D-positions to latitude/longitude
  note: select position
  path : Inport
  numPoses : Inport  Port=2
  originLLA : Inport  Port=3
  Constant : Constant  Value=zeros(1,100)
  Demux : Demux  Outputs=3
  MATLAB Function : MATLAB Function  TreatAsAtomicUnit=on
  Matrix Concatenate : Concatenate  Mode=Multidimensional array
  NED To LLA : AVE_Library/Essential/Transformation/NED To LLA
      settings: SourceProductName=AVE - Autonomous Vehicle Control Toolbox
  Reshape{,1..4} (5 alike) : Reshape  OutputDimensionality=Row vector (2-D)
  Selector : Selector  NumberOfDimensions=2  InputPortWidth=3  IndexOptions=Index vector (dialog),Select all  Indices=1,1  OutputSizes=1,1
  Selector1 : Selector  NumberOfDimensions=2  InputPortWidth=3  IndexOptions=Index vector (dialog),Select all  Indices=2,1  OutputSizes=1,1
  Terminator : Terminator
  assign position : Assignment  NumberOfDimensions=2  DiagnosticForDimensions=Warning  IndexOptions=Index vector (dialog),Assign all  Indices=1:2,1  OutputSizes=1,1
  posesOut : Outport
  wires:
  numPoses/1 -> MATLAB Function/2(numPoses)
  MATLAB Function/1(posesOut) -> posesOut/1
  Reshape4/1 -> NED To LLA/3
  Reshape3/1 -> NED To LLA/2
  Reshape2/1 -> NED To LLA/1
  Matrix Concatenate/1 -> assign position/2
  Demux/3 -> NED To LLA/6
  Demux/1 -> NED To LLA/4
  Demux/2 -> NED To LLA/5
  originLLA/1 -> Demux/1
  Constant/1 -> Reshape4/1
  Selector1/1 -> Reshape3/1
  Selector/1 -> Reshape2/1
  Reshape/1 -> Matrix Concatenate/1
  Reshape1/1 -> Matrix Concatenate/2
  NED To LLA/3 -> Terminator/1
  NED To LLA/2 -> Reshape1/1
  NED To LLA/1 -> Reshape/1
  assign position/1 -> MATLAB Function/1(posesIn)
  path/1 -> assign position/1, Selector1/1, Selector/1

== system MotionPlanner_Library/Asynchronous Motion Planner/make output struct/pulsed reset ==
  timestamp : Inport
  performedReset : Inport  Port=2
  AND : Logic  AllPortsSameDT=off  OutDataTypeStr=boolean
  Detect Change : simulink/Logic and Bit Operations/Detect Change  vinit=0  OutDataTypeStr=boolean
  reset : Outport
  wires:
  timestamp/1 -> Detect Change/1
  Detect Change/1 -> AND/1
  performedReset/1 -> AND/2
  AND/1 -> reset/1

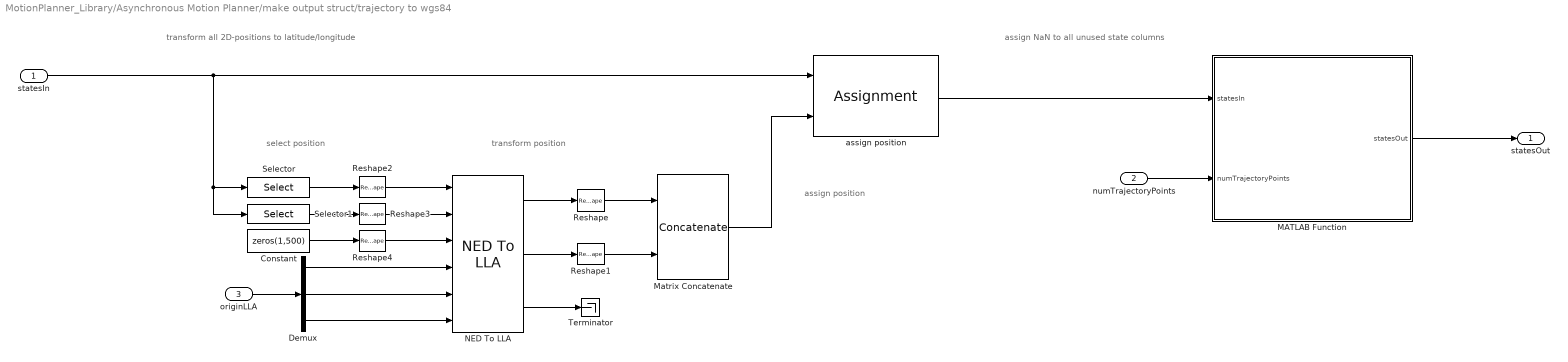
== system MotionPlanner_Library/Asynchronous Motion Planner/make output struct/trajectory to wgs84 ==
  note: select position
  note: transform all 2D-positions to latitude/longitude
  note: transform position
  note: assign position
  note: assign NaN to all unused state columns
  statesIn : Inport
  numTrajectoryPoints : Inport  Port=2
  originLLA : Inport  Port=3
  Constant : Constant  Value=zeros(1,500)
  Demux : Demux  Outputs=3
  MATLAB Function : MATLAB Function  TreatAsAtomicUnit=on
  Matrix Concatenate : Concatenate  Mode=Multidimensional array
  NED To LLA : AVE_Library/Essential/Transformation/NED To LLA
      settings: SourceProductName=AVE - Autonomous Vehicle Control Toolbox
  Reshape{,1..4} (5 alike) : Reshape  OutputDimensionality=Row vector (2-D)
  Selector : Selector  NumberOfDimensions=2  InputPortWidth=3  IndexOptions=Index vector (dialog),Select all  Indices=1,1  OutputSizes=1,1
  Selector1 : Selector  NumberOfDimensions=2  InputPortWidth=3  IndexOptions=Index vector (dialog),Select all  Indices=2,1  OutputSizes=1,1
  Terminator : Terminator
  assign position : Assignment  NumberOfDimensions=2  DiagnosticForDimensions=Warning  IndexOptions=Index vector (dialog),Assign all  Indices=1:2,1  OutputSizes=1,1
  statesOut : Outport
  wires:
  statesIn/1 -> Selector/1, Selector1/1, assign position/1
  assign position/1 -> MATLAB Function/1(statesIn)
  NED To LLA/1 -> Reshape/1
  NED To LLA/2 -> Reshape1/1
  NED To LLA/3 -> Terminator/1
  Reshape1/1 -> Matrix Concatenate/2
  Reshape/1 -> Matrix Concatenate/1
  Selector/1 -> Reshape2/1
  Selector1/1 -> Reshape3/1
  Constant/1 -> Reshape4/1
  originLLA/1 -> Demux/1
  Demux/2 -> NED To LLA/5
  Demux/1 -> NED To LLA/4
  Demux/3 -> NED To LLA/6
  Matrix Concatenate/1 -> assign position/2
  Reshape2/1 -> NED To LLA/1
  Reshape3/1 -> NED To LLA/2
  Reshape4/1 -> NED To LLA/3
  MATLAB Function/1(statesOut) -> statesOut/1
  numTrajectoryPoints/1 -> MATLAB Function/2(numTrajectoryPoints)

== matlab function MotionPlanner_Library/Asynchronous Motion Planner/Asynchronous Motion Planner/MATLAB Function ==
  data: trajNotInTime input; errorCodeInput input; errorCode output; errorCodeParameter input; plannerDisabled input; infeasibleProblem input
function errorCode = make_error_code(trajNotInTime, errorCodeInput, errorCodeParameter, plannerDisabled, infeasibleProblem)
    errorCode = uint8(0);
    if(errorCodeInput)
        errorCode = errorCodeInput;
    elseif(errorCodeParameter)
        errorCode = errorCodeParameter;
    elseif(plannerDisabled)
        errorCode = uint8(255);
    elseif(infeasibleProblem)
        errorCode = uint8(100);
    elseif(trajNotInTime)
        errorCode = uint8(200);
    end
end

== matlab function MotionPlanner_Library/Asynchronous Motion Planner/Planning Problem Generator/to cartesian obstacles/add_matlab ==
  data: u1 input; y output; u2 input
function y = add_matlab(u1, u2)
    y = u1 + u2;
end

== matlab function MotionPlanner_Library/Asynchronous Motion Planner/make output struct/trajectory to wgs84/MATLAB Function ==
  data: statesIn input; statesOut output; numTrajectoryPoints input
function statesOut = UnusedToNaN(statesIn, numTrajectoryPoints)
    statesOut = statesIn;
    maxPoints = size(statesIn, 2);
    if(numTrajectoryPoints < maxPoints)
        statesOut(:,(numTrajectoryPoints+1):end) = NaN;
    end
end

== matlab function MotionPlanner_Library/Asynchronous Motion Planner/make output struct/path to wgs84/MATLAB Function ==
  data: posesIn input; posesOut output; numPoses input
function posesOut = UnusedToNaN(posesIn, numPoses)
    posesOut = posesIn;
    maxPoints = size(posesIn, 2);
    if(numPoses < maxPoints)
        posesOut(:,(numPoses+1):end) = NaN;
    end
end
